simulink model "PLL__1"  (R2015a)
settings: Solver=ode45  StartTime=0.0  StopTime=10.0  RelTol=1e-3
values from neighbouring files (symbols this model uses):
  denC = [1 0]    [PLL_1.m]    (also in PLL_2.m; PLL_3.m)
  F_ref = 0    [PLL_1.m]    (also in PLL_2.m; PLL_3.m)
  G0 = 1e3    (= 1000)    [PLL_1.m]    (also in PLL_2.m; PLL_3.m)
  N = 10    [PLL_1.m]    (also in PLL_2.m; PLL_3.m)
  nomC = Vm    (= 10)    [PLL_1.m]    (also in PLL_2.m; PLL_3.m)
  RC = 2e-4    (= 0.0002)    [PLL_1.m]    (also in PLL_2.m; PLL_3.m)
  tau = 5e-5    (= 5e-05)    [PLL_1.m]    (also in PLL_2.m; PLL_3.m)
settings Model: Creator=mserrari  LastModifiedBy=mserrari

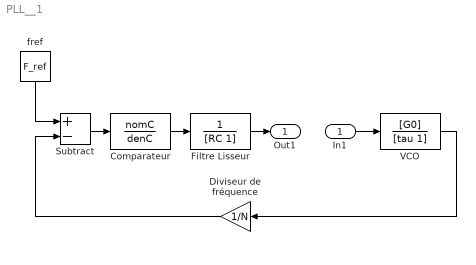
== system PLL__1 ==
  In1 : Inport
  Comparateur : TransferFcn  Numerator=nomC  Denominator=denC
  Diviseur de fréquence : Gain  Gain=1/N
  Filtre Lisseur : TransferFcn  Denominator=[RC 1]
  Subtract : Sum  Inputs=+-
  VCO : TransferFcn  Numerator=[G0]  Denominator=[tau 1]
  fref : Constant  Value=F_ref
  Out1 : Outport
  wires:
  Filtre Lisseur/1 -> Out1/1
  In1/1 -> VCO/1
  Comparateur/1 -> Filtre Lisseur/1
  Subtract/1 -> Comparateur/1
  VCO/1 -> Diviseur de fréquence/1
  Diviseur de fréquence/1 -> Subtract/2
  fref/1 -> Subtract/1
